simulink model "hpt_v2_1to1_switchlevel"  (R2025a)
settings: Solver=ode23tb  StartTime=0.0  StopTime=0.2  RelTol=1e-3
model workspace (MAT data in the model file):
  hpt_ctrl_Ts = 2e-05
  hpt_energy_bridge_polarity = -1
  hpt_energy_control_sign = -1
  hpt_energy_i_ki = 100
  hpt_energy_i_kp = 0.5
  hpt_energy_id_max = 20
  hpt_energy_openloop_amp = 0
  hpt_energy_openloop_phase = 0
  hpt_energy_vff_gain = 1.06
  hpt_grid_f0 = 50
  hpt_inj_phase_offset = -1.05
  hpt_m_energy = 0
  hpt_m_energy_max = 0.95
  hpt_m_reg = 0.1
  hpt_m_reg_max = 0.8
  hpt_pll_ki = 2500
  hpt_pll_kp = 80
  hpt_pwm_fs = 2000
  hpt_sac_actor_select_mode = 0
  hpt_sac_dynamic_reg_limit = 0.8
  hpt_sac_enable = 0
  hpt_sac_energy_enable = 0
  hpt_sac_energy_max = 0.95
  hpt_sac_fixed_energy_d = 0
  hpt_sac_fixed_energy_q = 0
  hpt_sac_fixed_reg_d = 0
  hpt_sac_fixed_reg_q = 0
  hpt_sac_guard_enable = 0
  hpt_sac_i_base_peak = 816.496580928
  hpt_sac_policy_mode = 0
  hpt_sac_reg_d_gain = 1
  hpt_sac_reg_max = 0.8
  hpt_sac_reg_polarity = 1
  hpt_sac_reg_q_gain = 0
  hpt_sac_topology_id = 1
  hpt_sac_vdc_ref = 800
  hpt_sac_vref_phase = 230
  hpt_swell_gain_scale = 1
  hpt_vdc_ki = 0.2
  hpt_vdc_kp = 0.1
  hpt_vdc_ref = 800
  hpt_vref_lv = 207
  hpt_vreg_ki = 0
  hpt_vreg_kp = 20
libraries: simulink x9, spsLinearTransformerLib x9, spsUniversalBridgeLib x4, spsGroundLib x4, spsThreePhaseVIMeasurementLib x3, spsSeriesRLCBranchLib x2, spsThreePhaseSeriesRLCBranchLib x2, spsIGBTLib x1, spsThreePhaseSourceLib x1, spsThreePhaseSeriesRLCLoadLib x1, spsVoltageMeasurementLib x1, spspowerguiLib x1
settings Model: Creator=m1391  LastModifiedBy=m1391

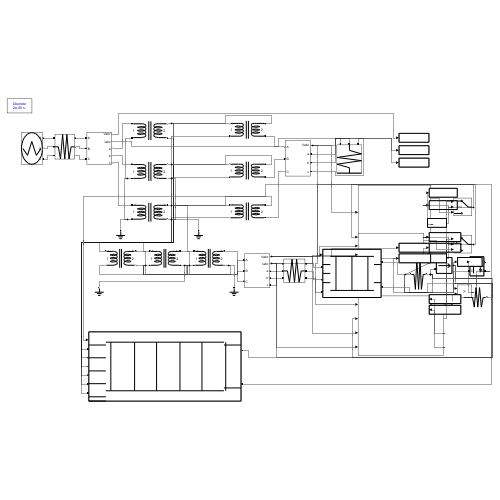
[thumbnail: Simulink's stored preview of the top-level diagram]
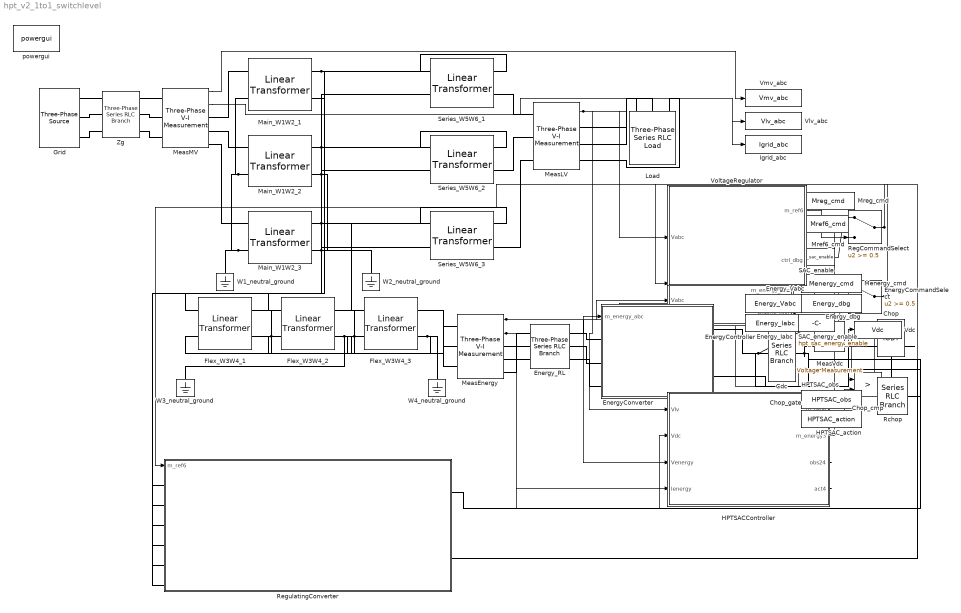
== system hpt_v2_1to1_switchlevel ==
  Cdc : spsSeriesRLCBranchLib/Series RLC Branch  LConnTagsString=__new0  RConnTagsString=__new0  BranchType=C  Resistance=1  Inductance=1e-3  SetiL0=off  InitialCurrent=0  Capacitance=0.0022  Setx0=on  InitialVoltage=800  Measurements=None
  Chop : spsIGBTLib/IGBT  Ron=0.001  Lon=0  Vf=1  Tf=1e-6  Tt=2e-6  IC=0  Rs=1e5  Cs=inf  Measurements=on
  Chop_cmp : RelationalOperator  Operator=>  OutDataTypeStr=boolean  RndMeth=Simplest  InputSameDT=off
  Chop_gate : Constant  Value=850
      mask Display: plot([20 80 80 20 20],[30 30 70 70 30]);
  EnergyCommandSelect : Switch  Threshold=0.5  SaturateOnIntegerOverflow=off  InputSameDT=off
  EnergyController : Subsystem
  EnergyConverter : Subsystem
      mask Display:
      | color('black');
      | plot([10 90 90 10 10],[10 10 90 90 10]);
      | plot([20 80],[78 78]); plot([20 80],[22 22]);
      | plot([28 28],[22 78]); plot([50 50],[22 78]); plot([72 72],[22 78]);
      | plot([10 20],[65 65]); plot([10 20],[50 50]); plot([10 20],[35 35]);
      | plot([80 90],[65 65]); plot([80 90],[35 35]);
  Energy_Iabc : ToWorkspace  VariableName=Energy_Iabc  SampleTime=2e-05
      mask Display: plot([10 90 90 10 10],[25 25 75 75 25]);
  Energy_RL : spsThreePhaseSeriesRLCBranchLib/Three-Phase Series RLC Branch  LConnTagsString=A|B|C  RConnTagsString=A|B|C  BranchType=RL  Resistance=0.05  Inductance=0.003  Capacitance=1e-6  Measurements=None
  Energy_Vabc : ToWorkspace  VariableName=Energy_Vabc  SampleTime=2e-05
      mask Display: plot([10 90 90 10 10],[25 25 75 75 25]);
  Energy_dbg : ToWorkspace  VariableName=Energy_dbg  SampleTime=2e-05
      mask Display: plot([10 90 90 10 10],[25 25 75 75 25]);
  Flex_W3W4_1 : spsLinearTransformerLib/Linear Transformer  UNITS=pu  NominalPower=[40000,50]  winding1=[230.9401,0.005,0.02]  winding2=[230.9401,0.005,0.02]  ThreeWindings=off  winding3=[ 315e3 0.002 0.08 ]  RmLm=[ 500 500 ]  Measurements=None  DataType=off
  Flex_W3W4_2 : spsLinearTransformerLib/Linear Transformer  UNITS=pu  NominalPower=[40000,50]  winding1=[230.9401,0.005,0.02]  winding2=[230.9401,0.005,0.02]  ThreeWindings=off  winding3=[ 315e3 0.002 0.08 ]  RmLm=[ 500 500 ]  Measurements=None  DataType=off
  Flex_W3W4_3 : spsLinearTransformerLib/Linear Transformer  UNITS=pu  NominalPower=[40000,50]  winding1=[230.9401,0.005,0.02]  winding2=[230.9401,0.005,0.02]  ThreeWindings=off  winding3=[ 315e3 0.002 0.08 ]  RmLm=[ 500 500 ]  Measurements=None  DataType=off
  Grid : spsThreePhaseSourceLib/Three-Phase Source  InternalConnection=Yg  VoltagePhases=off  Voltage=10000  PhaseAngle=0  Voltage_phases=[25e3 25e3 25e3]/sqrt(3)  PhaseAngles_phases=[0 -120 +120]  Frequency=50  NonIdealSource=on  SpecifyImpedance=off  Resistance=1e-3  Inductance=1e-5  ShortCircuitLevel=100e6  BaseVoltage=25e3  XRratio=7  BusType=swing  Pref=10e3  Qref=0  Prefabc=[10e3, 10e3, 10e3]  Qrefabc=[0, 0, 0]  Qmin=-inf  Qmax=inf
  HPTSACController : Subsystem
  HPTSAC_action : ToWorkspace  VariableName=HPTSAC_action  SampleTime=2e-05
      mask Display: plot([10 90 90 10 10],[25 25 75 75 25]);
  HPTSAC_obs : ToWorkspace  VariableName=HPTSAC_obs  SampleTime=2e-05
      mask Display: plot([10 90 90 10 10],[25 25 75 75 25]);
  Igrid_abc : ToWorkspace  VariableName=Igrid_abc  SampleTime=2e-05
      mask Display: plot([10 90 90 10 10],[25 25 75 75 25]);
  Load : spsThreePhaseSeriesRLCLoadLib/Three-Phase Series RLC Load  LConnTagsString=A|B|C  Configuration=Y (grounded)  NominalVoltage=400  Vabc=[1e3 1e3 1e3]  Vabcp=[1e3 1e3 1e3]  NominalFrequency=50  UnbalancedPower=off  ActivePower=400000  InductivePower=0  CapacitivePower=0  Pabc=[10e3 9e3 11e3]  QLabc=[100 90 110]  QCabc=[100 90 110]  Pabcp=[10e3 9e3 11e3]  QLabcp=[100 90 110]  QCabcp=[100 90 110]  Measurements=None  LoadType=constant Z
  Main_W1W2_1 : spsLinearTransformerLib/Linear Transformer  UNITS=pu  NominalPower=[133333.3333,50]  winding1=[5773.5027,0.005,0.025]  winding2=[230.9401,0.005,0.025]  ThreeWindings=off  winding3=[ 315e3 0.002 0.08 ]  RmLm=[ 500 500 ]  Measurements=None  DataType=off
  Main_W1W2_2 : spsLinearTransformerLib/Linear Transformer  UNITS=pu  NominalPower=[133333.3333,50]  winding1=[5773.5027,0.005,0.025]  winding2=[230.9401,0.005,0.025]  ThreeWindings=off  winding3=[ 315e3 0.002 0.08 ]  RmLm=[ 500 500 ]  Measurements=None  DataType=off
  Main_W1W2_3 : spsLinearTransformerLib/Linear Transformer  UNITS=pu  NominalPower=[133333.3333,50]  winding1=[5773.5027,0.005,0.025]  winding2=[230.9401,0.005,0.025]  ThreeWindings=off  winding3=[ 315e3 0.002 0.08 ]  RmLm=[ 500 500 ]  Measurements=None  DataType=off
  MeasEnergy : spsThreePhaseVIMeasurementLib/Three-Phase V-I Measurement  VoltageMeasurement=phase-to-ground  SetLabelV=off  LabelV=Vabc  Vpu=off  VpuLL=off  CurrentMeasurement=yes  SetLabelI=off  LabelI=Iabc  Ipu=off  Pbase=100e6  Vbase=500e3  OutputType=Complex  PhasorSimulation=off  PSBequivalent=0
  MeasLV : spsThreePhaseVIMeasurementLib/Three-Phase V-I Measurement  VoltageMeasurement=phase-to-ground  SetLabelV=off  LabelV=Vabc  Vpu=off  VpuLL=off  CurrentMeasurement=no  SetLabelI=off  LabelI=Iabc  Ipu=off  Pbase=100e6  Vbase=500e3  OutputType=Complex  PhasorSimulation=off  PSBequivalent=0
  MeasMV : spsThreePhaseVIMeasurementLib/Three-Phase V-I Measurement  VoltageMeasurement=phase-to-ground  SetLabelV=off  LabelV=Vabc  Vpu=off  VpuLL=off  CurrentMeasurement=yes  SetLabelI=off  LabelI=Iabc  Ipu=off  Pbase=100e6  Vbase=500e3  OutputType=Complex  PhasorSimulation=off  PSBequivalent=0
  MeasVdc : spsVoltageMeasurementLib/Voltage Measurement  PhasorSimulation=off  OutputType=Complex  PSBequivalent=0
  Menergy_cmd : ToWorkspace  VariableName=Menergy_cmd  SampleTime=2e-05
      mask Display: plot([10 90 90 10 10],[25 25 75 75 25]);
  Mref6_cmd : ToWorkspace  VariableName=Mref6_cmd  SampleTime=2e-05
      mask Display: plot([10 90 90 10 10],[25 25 75 75 25]);
  Mreg_cmd : ToWorkspace  VariableName=Mreg_cmd  SampleTime=2e-05
      mask Display: plot([10 90 90 10 10],[25 25 75 75 25]);
  Rchop : spsSeriesRLCBranchLib/Series RLC Branch  LConnTagsString=__new0  RConnTagsString=__new0  BranchType=R  Resistance=5.3333  Inductance=1e-3  SetiL0=off  InitialCurrent=0  Capacitance=1e-6  Setx0=off  InitialVoltage=0  Measurements=None
  RegCommandSelect : Switch  Threshold=0.5  SaturateOnIntegerOverflow=off  InputSameDT=off
  RegulatingConverter : Subsystem
      mask Display:
      | color('black');
      | plot([5 95 95 5 5],[10 10 90 90 10]);
      | plot([15 85],[78 78]); plot([15 85],[22 22]);
      | plot([18 18],[22 78]); plot([32 32],[22 78]);
      | plot([45 45],[22 78]); plot([59 59],[22 78]);
      | plot([72 72],[22 78]); plot([86 86],[22 78]);
      | plot([5 15],[75 75]); plot([5 15],[60 60]); plot([5 15],[45 45]);
      | plot([5 15],[30 30]); plot([5 15],[15 15]); plot([5 15],[10 10]);
      | plot([85 95],[75 75]); plot([85 95],[25 25]);
  SAC_enable : Constant  Value=hpt_sac_enable
      mask Display: plot([20 80 80 20 20],[30 30 70 70 30]);
  SAC_energy_enable : Constant  Value=hpt_sac_energy_enable
      mask Display: plot([20 80 80 20 20],[30 30 70 70 30]);
  Series_W5W6_1 : spsLinearTransformerLib/Linear Transformer  UNITS=pu  NominalPower=[30000,50]  winding1=[400,0.002,0.03]  winding2=[100,0.002,0.03]  ThreeWindings=off  winding3=[ 315e3 0.002 0.08 ]  RmLm=[ 500 500 ]  Measurements=None  DataType=off
  Series_W5W6_2 : spsLinearTransformerLib/Linear Transformer  UNITS=pu  NominalPower=[30000,50]  winding1=[400,0.002,0.03]  winding2=[100,0.002,0.03]  ThreeWindings=off  winding3=[ 315e3 0.002 0.08 ]  RmLm=[ 500 500 ]  Measurements=None  DataType=off
  Series_W5W6_3 : spsLinearTransformerLib/Linear Transformer  UNITS=pu  NominalPower=[30000,50]  winding1=[400,0.002,0.03]  winding2=[100,0.002,0.03]  ThreeWindings=off  winding3=[ 315e3 0.002 0.08 ]  RmLm=[ 500 500 ]  Measurements=None  DataType=off
  Vdc : ToWorkspace  VariableName=Vdc  SampleTime=2e-05
      mask Display: plot([10 90 90 10 10],[25 25 75 75 25]);
  Vlv_abc : ToWorkspace  VariableName=Vlv_abc  SampleTime=2e-05
      mask Display: plot([10 90 90 10 10],[25 25 75 75 25]);
  Vmv_abc : ToWorkspace  VariableName=Vmv_abc  SampleTime=2e-05
      mask Display: plot([10 90 90 10 10],[25 25 75 75 25]);
  VoltageRegulator : Subsystem
  W1_neutral_ground : spsGroundLib/Ground  LConnTagsString=a
  W2_neutral_ground : spsGroundLib/Ground  LConnTagsString=a
  W3_neutral_ground : spsGroundLib/Ground  LConnTagsString=a
  W4_neutral_ground : spsGroundLib/Ground  LConnTagsString=a
  Zg : spsThreePhaseSeriesRLCBranchLib/Three-Phase Series RLC Branch  LConnTagsString=A|B|C  RConnTagsString=A|B|C  BranchType=RL  Resistance=11.7851  Inductance=0.26259  Capacitance=1e-6  Measurements=None
  powergui : spspowerguiLib/powergui  Priority=1  SimulationMode=Discrete  SampleTime=2e-05  frequency=60  Iterations=50  frequencyindice=60  Pbase=100e6  ErrMax=1e-4  UnitsV=kV  UnitsW=MW  buscounter=0  FunctionMessages=off  echomessages=off  EnableUseOfTLC=off  CurrentSourceSwitches=off  DisableSnubberDevices=off  DisableRonSwitches=off  DisableVfSwitches=off  DisplayEquations=off  AutomaticDiscreteSolvers=off  SolverType=Tustin/Backward Euler (TBE)  Interpol=off  ExternalGateDelay=off  methode=off  Ts=100  x0status=blocks  SPID=on  SwTol=0  HookPort=off  NonlinearTolerance=1e-4  nMaxIteration=100  ContinueOnMaxIteration=off  RestoreLinks=warning  ResistiveCurrentMeasurement=off  Frange=[0:2:500]  Ylog=off  Xlog=on  ShowGrid=off  save=off  variable=ZData  structure=0  ZoomFFT=off  StartTime=0.0  cycles=1  DisplayStyle=1  fundamental=60  FreqAxis=off  MaxFrequency=1000  frequencyindicesteady=1  RmsSteady=1  display=off
  wires:
  MeasVdc/1 -> Chop_cmp/1, Vdc/1, HPTSACController/2(Vdc), EnergyController/1(Vdc)
  Chop_gate/1 -> Chop_cmp/2
  Chop_cmp/1 -> Chop/1
  MeasMV/1 -> Vmv_abc/1
  MeasMV/2 -> Igrid_abc/1
  MeasLV/1 -> Vlv_abc/1, VoltageRegulator/1(Vabc), HPTSACController/1(Vlv)
  VoltageRegulator/1(m_ref6) -> RegCommandSelect/3
  HPTSACController/1(m_reg6) -> RegCommandSelect/1
  SAC_enable/1 -> RegCommandSelect/2
  RegCommandSelect/1 -> RegulatingConverter/1(m_ref6), Mref6_cmd/1
  VoltageRegulator/2(ctrl_dbg) -> Mreg_cmd/1
  MeasEnergy/1 -> EnergyController/2(Vabc), HPTSACController/3(Venergy), Energy_Vabc/1
  MeasEnergy/2 -> EnergyController/3(Iabc), HPTSACController/4(Ienergy), Energy_Iabc/1
  EnergyController/1(m_energy_abc) -> EnergyCommandSelect/3
  HPTSACController/2(m_energy3) -> EnergyCommandSelect/1
  SAC_energy_enable/1 -> EnergyCommandSelect/2
  EnergyCommandSelect/1 -> EnergyConverter/1(m_energy_abc), Menergy_cmd/1
  EnergyController/2(energy_dbg) -> Energy_dbg/1
  HPTSACController/3(obs24) -> HPTSAC_obs/1
  HPTSACController/4(act4) -> HPTSAC_action/1
  connections:
  Grid/RConn1 -- Zg/LConn1
  Zg/RConn1 -- MeasMV/LConn1
  MeasMV/RConn1 -- Main_W1W2_1/LConn1
  Series_W5W6_1/RConn1 -- Main_W1W2_1/RConn1 -- Flex_W3W4_1/LConn1
  Series_W5W6_1/RConn2 -- MeasLV/LConn1
  MeasLV/RConn1 -- Load/LConn1
  Flex_W3W4_1/RConn1 -- MeasEnergy/LConn1
  MeasEnergy/RConn1 -- Energy_RL/LConn1
  Energy_RL/RConn1 -- EnergyConverter/LConn1
  Series_W5W6_1/LConn1 -- RegulatingConverter/LConn1
  Series_W5W6_1/LConn2 -- RegulatingConverter/LConn2
  Grid/RConn2 -- Zg/LConn2
  Zg/RConn2 -- MeasMV/LConn2
  MeasMV/RConn2 -- Main_W1W2_2/LConn1
  Series_W5W6_2/RConn1 -- Main_W1W2_2/RConn1 -- Flex_W3W4_2/LConn1
  Series_W5W6_2/RConn2 -- MeasLV/LConn2
  MeasLV/RConn2 -- Load/LConn2
  Flex_W3W4_2/RConn1 -- MeasEnergy/LConn2
  MeasEnergy/RConn2 -- Energy_RL/LConn2
  Energy_RL/RConn2 -- EnergyConverter/LConn2
  Series_W5W6_2/LConn1 -- RegulatingConverter/LConn3
  Series_W5W6_2/LConn2 -- RegulatingConverter/LConn4
  Grid/RConn3 -- Zg/LConn3
  Zg/RConn3 -- MeasMV/LConn3
  MeasMV/RConn3 -- Main_W1W2_3/LConn1
  Series_W5W6_3/RConn1 -- Main_W1W2_3/RConn1 -- Flex_W3W4_3/LConn1
  Series_W5W6_3/RConn2 -- MeasLV/LConn3
  MeasLV/RConn3 -- Load/LConn3
  Flex_W3W4_3/RConn1 -- MeasEnergy/LConn3
  MeasEnergy/RConn3 -- Energy_RL/LConn3
  Energy_RL/RConn3 -- EnergyConverter/LConn3
  Series_W5W6_3/LConn1 -- RegulatingConverter/LConn5
  Series_W5W6_3/LConn2 -- RegulatingConverter/LConn6
  Main_W1W2_2/LConn2 -- Main_W1W2_1/LConn2 -- Main_W1W2_3/LConn2 -- W1_neutral_ground/LConn1
  Main_W1W2_2/RConn2 -- Main_W1W2_1/RConn2 -- Main_W1W2_3/RConn2 -- W2_neutral_ground/LConn1
  Flex_W3W4_2/LConn2 -- Flex_W3W4_1/LConn2 -- Flex_W3W4_3/LConn2 -- W3_neutral_ground/LConn1
  Flex_W3W4_2/RConn2 -- Flex_W3W4_1/RConn2 -- Flex_W3W4_3/RConn2 -- W4_neutral_ground/LConn1
  EnergyConverter/RConn1 -- Cdc/LConn1 -- RegulatingConverter/RConn1 -- MeasVdc/LConn1 -- Chop/LConn1
  EnergyConverter/RConn2 -- RegulatingConverter/RConn2 -- MeasVdc/LConn2 -- Cdc/RConn1 -- Rchop/RConn1
  Chop/RConn1 -- Rchop/LConn1

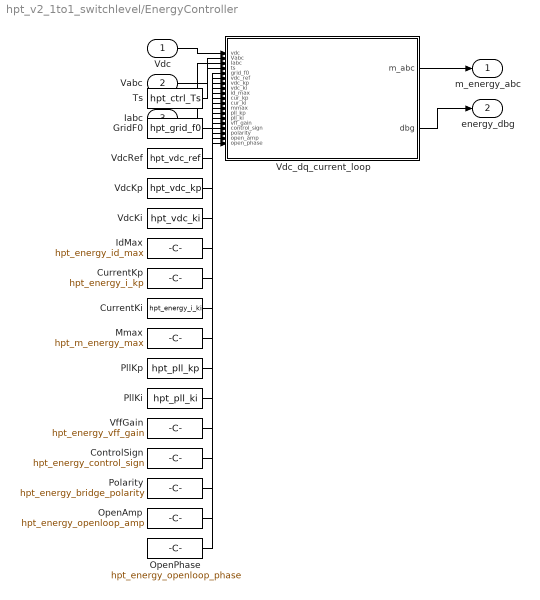
== system hpt_v2_1to1_switchlevel/EnergyController ==
  Vdc : Inport
  Vabc : Inport  Port=2
  Iabc : Inport  Port=3
  ControlSign : Constant  Value=hpt_energy_control_sign
      mask Display: plot([20 80 80 20 20],[30 30 70 70 30]);
  CurrentKi : Constant  Value=hpt_energy_i_ki
      mask Display: plot([20 80 80 20 20],[30 30 70 70 30]);
  CurrentKp : Constant  Value=hpt_energy_i_kp
      mask Display: plot([20 80 80 20 20],[30 30 70 70 30]);
  GridF0 : Constant  Value=hpt_grid_f0
      mask Display: plot([20 80 80 20 20],[30 30 70 70 30]);
  IdMax : Constant  Value=hpt_energy_id_max
      mask Display: plot([20 80 80 20 20],[30 30 70 70 30]);
  Mmax : Constant  Value=hpt_m_energy_max
      mask Display: plot([20 80 80 20 20],[30 30 70 70 30]);
  OpenAmp : Constant  Value=hpt_energy_openloop_amp
      mask Display: plot([20 80 80 20 20],[30 30 70 70 30]);
  OpenPhase : Constant  Value=hpt_energy_openloop_phase
      mask Display: plot([20 80 80 20 20],[30 30 70 70 30]);
  PllKi : Constant  Value=hpt_pll_ki
      mask Display: plot([20 80 80 20 20],[30 30 70 70 30]);
  PllKp : Constant  Value=hpt_pll_kp
      mask Display: plot([20 80 80 20 20],[30 30 70 70 30]);
  Polarity : Constant  Value=hpt_energy_bridge_polarity
      mask Display: plot([20 80 80 20 20],[30 30 70 70 30]);
  Ts : Constant  Value=hpt_ctrl_Ts
      mask Display: plot([20 80 80 20 20],[30 30 70 70 30]);
  VdcKi : Constant  Value=hpt_vdc_ki
      mask Display: plot([20 80 80 20 20],[30 30 70 70 30]);
  VdcKp : Constant  Value=hpt_vdc_kp
      mask Display: plot([20 80 80 20 20],[30 30 70 70 30]);
  VdcRef : Constant  Value=hpt_vdc_ref
      mask Display: plot([20 80 80 20 20],[30 30 70 70 30]);
  Vdc_dq_current_loop : MATLAB Function  TreatAsAtomicUnit=on
  VffGain : Constant  Value=hpt_energy_vff_gain
      mask Display: plot([20 80 80 20 20],[30 30 70 70 30]);
  m_energy_abc : Outport
  energy_dbg : Outport  Port=2
  wires:
  Ts/1 -> Vdc_dq_current_loop/4(ts)
  GridF0/1 -> Vdc_dq_current_loop/5(grid_f0)
  VdcRef/1 -> Vdc_dq_current_loop/6(vdc_ref)
  VdcKp/1 -> Vdc_dq_current_loop/7(vdc_kp)
  VdcKi/1 -> Vdc_dq_current_loop/8(vdc_ki)
  IdMax/1 -> Vdc_dq_current_loop/9(id_max)
  CurrentKp/1 -> Vdc_dq_current_loop/10(cur_kp)
  CurrentKi/1 -> Vdc_dq_current_loop/11(cur_ki)
  Mmax/1 -> Vdc_dq_current_loop/12(mmax)
  PllKp/1 -> Vdc_dq_current_loop/13(pll_kp)
  PllKi/1 -> Vdc_dq_current_loop/14(pll_ki)
  VffGain/1 -> Vdc_dq_current_loop/15(vff_gain)
  ControlSign/1 -> Vdc_dq_current_loop/16(control_sign)
  Polarity/1 -> Vdc_dq_current_loop/17(polarity)
  OpenAmp/1 -> Vdc_dq_current_loop/18(open_amp)
  OpenPhase/1 -> Vdc_dq_current_loop/19(open_phase)
  Vdc/1 -> Vdc_dq_current_loop/1(vdc)
  Vabc/1 -> Vdc_dq_current_loop/2(Vabc)
  Iabc/1 -> Vdc_dq_current_loop/3(Iabc)
  Vdc_dq_current_loop/1(m_abc) -> m_energy_abc/1
  Vdc_dq_current_loop/2(dbg) -> energy_dbg/1

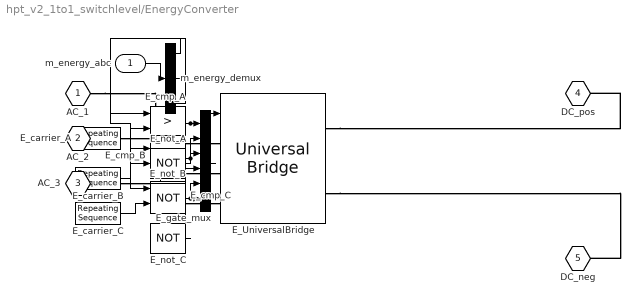
== system hpt_v2_1to1_switchlevel/EnergyConverter ==
  m_energy_abc : Inport
  E_UniversalBridge : spsUniversalBridgeLib/Universal Bridge  Arms=3  SnubberResistance=1e5  SnubberCapacitance=inf  Device=IGBT / Diodes  Ron=1e-3  Lon=0  ForwardVoltages=[0.8 0.8]  ForwardVoltage=0  GTOparameters=[ 10e-6 , 20e-6 ]  IGBTparameters=[ 1e-6 , 2e-6 ]  Measurements=None  Measurements_2=None  converterType=Rectifier
  E_carrier_A : simulink/Sources/Repeating Sequence  rep_seq_t=[0 0.5/hpt_pwm_fs 1/hpt_pwm_fs]  rep_seq_y=[-1 1 -1]
  E_carrier_B : simulink/Sources/Repeating Sequence  rep_seq_t=[0 0.5/hpt_pwm_fs 1/hpt_pwm_fs]  rep_seq_y=[-1 1 -1]
  E_carrier_C : simulink/Sources/Repeating Sequence  rep_seq_t=[0 0.5/hpt_pwm_fs 1/hpt_pwm_fs]  rep_seq_y=[-1 1 -1]
  E_cmp_A : RelationalOperator  Operator=>  OutDataTypeStr=boolean  RndMeth=Simplest  InputSameDT=off
  E_cmp_B : RelationalOperator  Operator=>  OutDataTypeStr=boolean  RndMeth=Simplest  InputSameDT=off
  E_cmp_C : RelationalOperator  Operator=>  OutDataTypeStr=boolean  RndMeth=Simplest  InputSameDT=off
  E_gate_mux : Mux  Inputs=6
  E_not_A : Logic  Operator=NOT  AllPortsSameDT=off  OutDataTypeStr=boolean
  E_not_B : Logic  Operator=NOT  AllPortsSameDT=off  OutDataTypeStr=boolean
  E_not_C : Logic  Operator=NOT  AllPortsSameDT=off  OutDataTypeStr=boolean
  m_energy_demux : Demux  Outputs=3
  AC_1 : PMIOPort  Side=Left
  AC_2 : PMIOPort  Port=2  Side=Left
  AC_3 : PMIOPort  Port=3  Side=Left
  DC_pos : PMIOPort  Port=4  Side=Right
  DC_neg : PMIOPort  Port=5  Side=Right
  wires:
  m_energy_abc/1 -> m_energy_demux/1
  m_energy_demux/1 -> E_cmp_A/1
  E_carrier_A/1 -> E_cmp_A/2
  E_cmp_A/1 -> E_gate_mux/1, E_not_A/1
  E_not_A/1 -> E_gate_mux/2
  m_energy_demux/2 -> E_cmp_B/1
  E_carrier_B/1 -> E_cmp_B/2
  E_cmp_B/1 -> E_gate_mux/3, E_not_B/1
  E_not_B/1 -> E_gate_mux/4
  m_energy_demux/3 -> E_cmp_C/1
  E_carrier_C/1 -> E_cmp_C/2
  E_cmp_C/1 -> E_gate_mux/5, E_not_C/1
  E_not_C/1 -> E_gate_mux/6
  E_gate_mux/1 -> E_UniversalBridge/1
  connections:
  AC_1/RConn1 -- E_UniversalBridge/LConn1
  AC_2/RConn1 -- E_UniversalBridge/LConn2
  AC_3/RConn1 -- E_UniversalBridge/LConn3
  E_UniversalBridge/RConn1 -- DC_pos/RConn1
  E_UniversalBridge/RConn2 -- DC_neg/RConn1

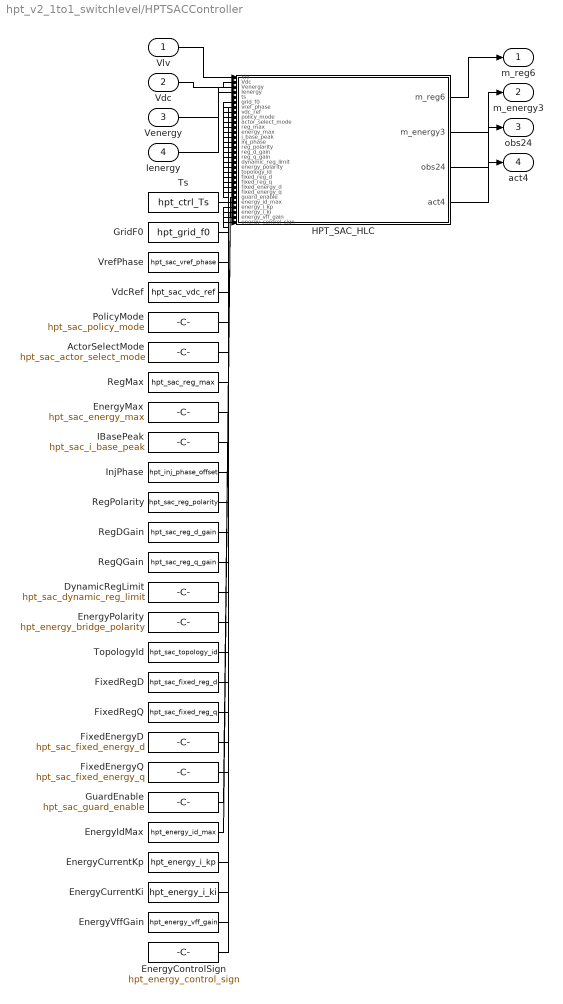
== system hpt_v2_1to1_switchlevel/HPTSACController ==
  Vlv : Inport
  Vdc : Inport  Port=2
  Venergy : Inport  Port=3
  Ienergy : Inport  Port=4
  ActorSelectMode : Constant  Value=hpt_sac_actor_select_mode
      mask Display: plot([20 80 80 20 20],[30 30 70 70 30]);
  DynamicRegLimit : Constant  Value=hpt_sac_dynamic_reg_limit
      mask Display: plot([20 80 80 20 20],[30 30 70 70 30]);
  EnergyControlSign : Constant  Value=hpt_energy_control_sign
      mask Display: plot([20 80 80 20 20],[30 30 70 70 30]);
  EnergyCurrentKi : Constant  Value=hpt_energy_i_ki
      mask Display: plot([20 80 80 20 20],[30 30 70 70 30]);
  EnergyCurrentKp : Constant  Value=hpt_energy_i_kp
      mask Display: plot([20 80 80 20 20],[30 30 70 70 30]);
  EnergyIdMax : Constant  Value=hpt_energy_id_max
      mask Display: plot([20 80 80 20 20],[30 30 70 70 30]);
  EnergyMax : Constant  Value=hpt_sac_energy_max
      mask Display: plot([20 80 80 20 20],[30 30 70 70 30]);
  EnergyPolarity : Constant  Value=hpt_energy_bridge_polarity
      mask Display: plot([20 80 80 20 20],[30 30 70 70 30]);
  EnergyVffGain : Constant  Value=hpt_energy_vff_gain
      mask Display: plot([20 80 80 20 20],[30 30 70 70 30]);
  FixedEnergyD : Constant  Value=hpt_sac_fixed_energy_d
      mask Display: plot([20 80 80 20 20],[30 30 70 70 30]);
  FixedEnergyQ : Constant  Value=hpt_sac_fixed_energy_q
      mask Display: plot([20 80 80 20 20],[30 30 70 70 30]);
  FixedRegD : Constant  Value=hpt_sac_fixed_reg_d
      mask Display: plot([20 80 80 20 20],[30 30 70 70 30]);
  FixedRegQ : Constant  Value=hpt_sac_fixed_reg_q
      mask Display: plot([20 80 80 20 20],[30 30 70 70 30]);
  GridF0 : Constant  Value=hpt_grid_f0
      mask Display: plot([20 80 80 20 20],[30 30 70 70 30]);
  GuardEnable : Constant  Value=hpt_sac_guard_enable
      mask Display: plot([20 80 80 20 20],[30 30 70 70 30]);
  HPT_SAC_HLC : MATLAB Function  TreatAsAtomicUnit=on
  IBasePeak : Constant  Value=hpt_sac_i_base_peak
      mask Display: plot([20 80 80 20 20],[30 30 70 70 30]);
  InjPhase : Constant  Value=hpt_inj_phase_offset
      mask Display: plot([20 80 80 20 20],[30 30 70 70 30]);
  PolicyMode : Constant  Value=hpt_sac_policy_mode
      mask Display: plot([20 80 80 20 20],[30 30 70 70 30]);
  RegDGain : Constant  Value=hpt_sac_reg_d_gain
      mask Display: plot([20 80 80 20 20],[30 30 70 70 30]);
  RegMax : Constant  Value=hpt_sac_reg_max
      mask Display: plot([20 80 80 20 20],[30 30 70 70 30]);
  RegPolarity : Constant  Value=hpt_sac_reg_polarity
      mask Display: plot([20 80 80 20 20],[30 30 70 70 30]);
  RegQGain : Constant  Value=hpt_sac_reg_q_gain
      mask Display: plot([20 80 80 20 20],[30 30 70 70 30]);
  TopologyId : Constant  Value=hpt_sac_topology_id
      mask Display: plot([20 80 80 20 20],[30 30 70 70 30]);
  Ts : Constant  Value=hpt_ctrl_Ts
      mask Display: plot([20 80 80 20 20],[30 30 70 70 30]);
  VdcRef : Constant  Value=hpt_sac_vdc_ref
      mask Display: plot([20 80 80 20 20],[30 30 70 70 30]);
  VrefPhase : Constant  Value=hpt_sac_vref_phase
      mask Display: plot([20 80 80 20 20],[30 30 70 70 30]);
  m_reg6 : Outport
  m_energy3 : Outport  Port=2
  obs24 : Outport  Port=3
  act4 : Outport  Port=4
  wires:
  Ts/1 -> HPT_SAC_HLC/5(ts)
  GridF0/1 -> HPT_SAC_HLC/6(grid_f0)
  VrefPhase/1 -> HPT_SAC_HLC/7(vref_phase)
  VdcRef/1 -> HPT_SAC_HLC/8(vdc_ref)
  PolicyMode/1 -> HPT_SAC_HLC/9(policy_mode)
  ActorSelectMode/1 -> HPT_SAC_HLC/10(actor_select_mode)
  RegMax/1 -> HPT_SAC_HLC/11(reg_max)
  EnergyMax/1 -> HPT_SAC_HLC/12(energy_max)
  IBasePeak/1 -> HPT_SAC_HLC/13(i_base_peak)
  InjPhase/1 -> HPT_SAC_HLC/14(inj_phase)
  RegPolarity/1 -> HPT_SAC_HLC/15(reg_polarity)
  RegDGain/1 -> HPT_SAC_HLC/16(reg_d_gain)
  RegQGain/1 -> HPT_SAC_HLC/17(reg_q_gain)
  DynamicRegLimit/1 -> HPT_SAC_HLC/18(dynamic_reg_limit)
  EnergyPolarity/1 -> HPT_SAC_HLC/19(energy_polarity)
  TopologyId/1 -> HPT_SAC_HLC/20(topology_id)
  FixedRegD/1 -> HPT_SAC_HLC/21(fixed_reg_d)
  FixedRegQ/1 -> HPT_SAC_HLC/22(fixed_reg_q)
  FixedEnergyD/1 -> HPT_SAC_HLC/23(fixed_energy_d)
  FixedEnergyQ/1 -> HPT_SAC_HLC/24(fixed_energy_q)
  GuardEnable/1 -> HPT_SAC_HLC/25(guard_enable)
  EnergyIdMax/1 -> HPT_SAC_HLC/26(energy_id_max)
  EnergyCurrentKp/1 -> HPT_SAC_HLC/27(energy_i_kp)
  EnergyCurrentKi/1 -> HPT_SAC_HLC/28(energy_i_ki)
  EnergyVffGain/1 -> HPT_SAC_HLC/29(energy_vff_gain)
  EnergyControlSign/1 -> HPT_SAC_HLC/30(energy_control_sign)
  Vlv/1 -> HPT_SAC_HLC/1(Vlv)
  Vdc/1 -> HPT_SAC_HLC/2(Vdc)
  Venergy/1 -> HPT_SAC_HLC/3(Venergy)
  Ienergy/1 -> HPT_SAC_HLC/4(Ienergy)
  HPT_SAC_HLC/1(m_reg6) -> m_reg6/1
  HPT_SAC_HLC/2(m_energy3) -> m_energy3/1
  HPT_SAC_HLC/3(obs24) -> obs24/1
  HPT_SAC_HLC/4(act4) -> act4/1

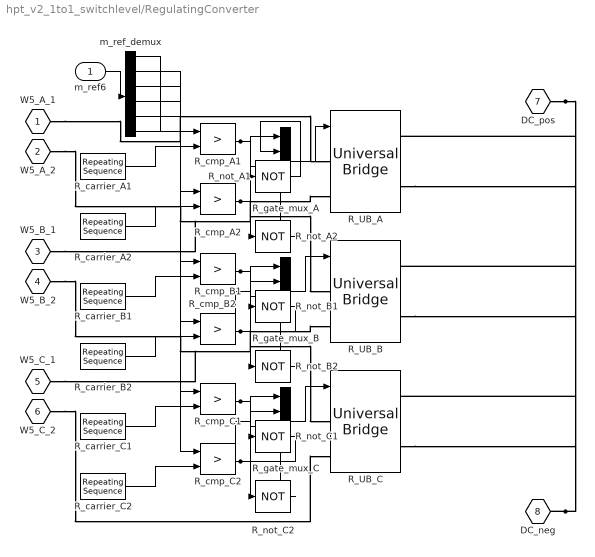
== system hpt_v2_1to1_switchlevel/RegulatingConverter ==
  m_ref6 : Inport
  R_UB_A : spsUniversalBridgeLib/Universal Bridge  Arms=2  SnubberResistance=1e5  SnubberCapacitance=1e-9  Device=IGBT / Diodes  Ron=1e-3  Lon=0  ForwardVoltages="[  0  0  ]"  ForwardVoltage=0  GTOparameters=[ 10e-6 , 20e-6 ]  IGBTparameters=[ 1e-6 , 2e-6 ]  Measurements=None  Measurements_2=None  converterType=Rectifier
  R_UB_B : spsUniversalBridgeLib/Universal Bridge  Arms=2  SnubberResistance=1e5  SnubberCapacitance=1e-9  Device=IGBT / Diodes  Ron=1e-3  Lon=0  ForwardVoltages="[  0  0  ]"  ForwardVoltage=0  GTOparameters=[ 10e-6 , 20e-6 ]  IGBTparameters=[ 1e-6 , 2e-6 ]  Measurements=None  Measurements_2=None  converterType=Rectifier
  R_UB_C : spsUniversalBridgeLib/Universal Bridge  Arms=2  SnubberResistance=1e5  SnubberCapacitance=1e-9  Device=IGBT / Diodes  Ron=1e-3  Lon=0  ForwardVoltages="[  0  0  ]"  ForwardVoltage=0  GTOparameters=[ 10e-6 , 20e-6 ]  IGBTparameters=[ 1e-6 , 2e-6 ]  Measurements=None  Measurements_2=None  converterType=Rectifier
  R_carrier_A1 : simulink/Sources/Repeating Sequence  rep_seq_t=[0 0.5/hpt_pwm_fs 1/hpt_pwm_fs]  rep_seq_y=[-1 1 -1]
  R_carrier_A2 : simulink/Sources/Repeating Sequence  rep_seq_t=[0 0.5/hpt_pwm_fs 1/hpt_pwm_fs]  rep_seq_y=[-1 1 -1]
  R_carrier_B1 : simulink/Sources/Repeating Sequence  rep_seq_t=[0 0.5/hpt_pwm_fs 1/hpt_pwm_fs]  rep_seq_y=[-1 1 -1]
  R_carrier_B2 : simulink/Sources/Repeating Sequence  rep_seq_t=[0 0.5/hpt_pwm_fs 1/hpt_pwm_fs]  rep_seq_y=[-1 1 -1]
  R_carrier_C1 : simulink/Sources/Repeating Sequence  rep_seq_t=[0 0.5/hpt_pwm_fs 1/hpt_pwm_fs]  rep_seq_y=[-1 1 -1]
  R_carrier_C2 : simulink/Sources/Repeating Sequence  rep_seq_t=[0 0.5/hpt_pwm_fs 1/hpt_pwm_fs]  rep_seq_y=[-1 1 -1]
  R_cmp_A1 : RelationalOperator  Operator=>  OutDataTypeStr=boolean  RndMeth=Simplest  InputSameDT=off
  R_cmp_A2 : RelationalOperator  Operator=>  OutDataTypeStr=boolean  RndMeth=Simplest  InputSameDT=off
  R_cmp_B1 : RelationalOperator  Operator=>  OutDataTypeStr=boolean  RndMeth=Simplest  InputSameDT=off
  R_cmp_B2 : RelationalOperator  Operator=>  OutDataTypeStr=boolean  RndMeth=Simplest  InputSameDT=off
  R_cmp_C1 : RelationalOperator  Operator=>  OutDataTypeStr=boolean  RndMeth=Simplest  InputSameDT=off
  R_cmp_C2 : RelationalOperator  Operator=>  OutDataTypeStr=boolean  RndMeth=Simplest  InputSameDT=off
  R_gate_mux_A : Mux
  R_gate_mux_B : Mux
  R_gate_mux_C : Mux
  R_not_A1 : Logic  Operator=NOT  AllPortsSameDT=off  OutDataTypeStr=boolean
  R_not_A2 : Logic  Operator=NOT  AllPortsSameDT=off  OutDataTypeStr=boolean
  R_not_B1 : Logic  Operator=NOT  AllPortsSameDT=off  OutDataTypeStr=boolean
  R_not_B2 : Logic  Operator=NOT  AllPortsSameDT=off  OutDataTypeStr=boolean
  R_not_C1 : Logic  Operator=NOT  AllPortsSameDT=off  OutDataTypeStr=boolean
  R_not_C2 : Logic  Operator=NOT  AllPortsSameDT=off  OutDataTypeStr=boolean
  m_ref_demux : Demux  Outputs=6
  W5_A_1 : PMIOPort  Side=Left
  W5_A_2 : PMIOPort  Port=2  Side=Left
  W5_B_1 : PMIOPort  Port=3  Side=Left
  W5_B_2 : PMIOPort  Port=4  Side=Left
  W5_C_1 : PMIOPort  Port=5  Side=Left
  W5_C_2 : PMIOPort  Port=6  Side=Left
  DC_pos : PMIOPort  Port=7  Side=Right
  DC_neg : PMIOPort  Port=8  Side=Right
  wires:
  m_ref6/1 -> m_ref_demux/1
  m_ref_demux/1 -> R_cmp_A1/1
  R_carrier_A1/1 -> R_cmp_A1/2
  R_cmp_A1/1 -> R_gate_mux_A/1, R_not_A1/1
  R_not_A1/1 -> R_gate_mux_A/2
  m_ref_demux/2 -> R_cmp_A2/1
  R_carrier_A2/1 -> R_cmp_A2/2
  R_cmp_A2/1 -> R_gate_mux_A/3, R_not_A2/1
  R_not_A2/1 -> R_gate_mux_A/4
  R_gate_mux_A/1 -> R_UB_A/1
  m_ref_demux/3 -> R_cmp_B1/1
  R_carrier_B1/1 -> R_cmp_B1/2
  R_cmp_B1/1 -> R_gate_mux_B/1, R_not_B1/1
  R_not_B1/1 -> R_gate_mux_B/2
  m_ref_demux/4 -> R_cmp_B2/1
  R_carrier_B2/1 -> R_cmp_B2/2
  R_cmp_B2/1 -> R_gate_mux_B/3, R_not_B2/1
  R_not_B2/1 -> R_gate_mux_B/4
  R_gate_mux_B/1 -> R_UB_B/1
  m_ref_demux/5 -> R_cmp_C1/1
  R_carrier_C1/1 -> R_cmp_C1/2
  R_cmp_C1/1 -> R_gate_mux_C/1, R_not_C1/1
  R_not_C1/1 -> R_gate_mux_C/2
  m_ref_demux/6 -> R_cmp_C2/1
  R_carrier_C2/1 -> R_cmp_C2/2
  R_cmp_C2/1 -> R_gate_mux_C/3, R_not_C2/1
  R_not_C2/1 -> R_gate_mux_C/4
  R_gate_mux_C/1 -> R_UB_C/1
  connections:
  W5_A_1/RConn1 -- R_UB_A/LConn1
  W5_A_2/RConn1 -- R_UB_A/LConn2
  W5_B_1/RConn1 -- R_UB_B/LConn1
  W5_B_2/RConn1 -- R_UB_B/LConn2
  W5_C_1/RConn1 -- R_UB_C/LConn1
  W5_C_2/RConn1 -- R_UB_C/LConn2
  R_UB_A/RConn1 -- DC_pos/RConn1 -- R_UB_B/RConn1 -- R_UB_C/RConn1
  R_UB_A/RConn2 -- R_UB_B/RConn2 -- DC_neg/RConn1 -- R_UB_C/RConn2

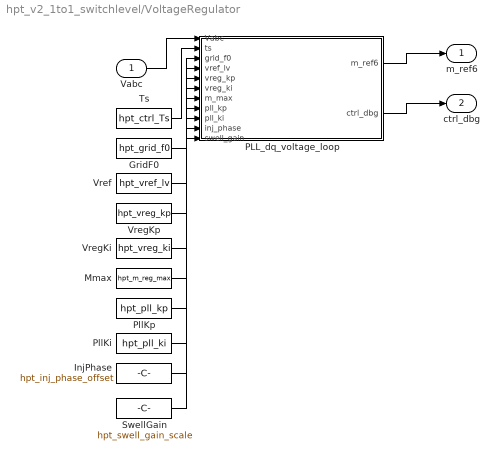
== system hpt_v2_1to1_switchlevel/VoltageRegulator ==
  Vabc : Inport
  GridF0 : Constant  Value=hpt_grid_f0
      mask Display: plot([20 80 80 20 20],[30 30 70 70 30]);
  InjPhase : Constant  Value=hpt_inj_phase_offset
      mask Display: plot([20 80 80 20 20],[30 30 70 70 30]);
  Mmax : Constant  Value=hpt_m_reg_max
      mask Display: plot([20 80 80 20 20],[30 30 70 70 30]);
  PLL_dq_voltage_loop : MATLAB Function  TreatAsAtomicUnit=on
  PllKi : Constant  Value=hpt_pll_ki
      mask Display: plot([20 80 80 20 20],[30 30 70 70 30]);
  PllKp : Constant  Value=hpt_pll_kp
      mask Display: plot([20 80 80 20 20],[30 30 70 70 30]);
  SwellGain : Constant  Value=hpt_swell_gain_scale
      mask Display: plot([20 80 80 20 20],[30 30 70 70 30]);
  Ts : Constant  Value=hpt_ctrl_Ts
      mask Display: plot([20 80 80 20 20],[30 30 70 70 30]);
  Vref : Constant  Value=hpt_vref_lv
      mask Display: plot([20 80 80 20 20],[30 30 70 70 30]);
  VregKi : Constant  Value=hpt_vreg_ki
      mask Display: plot([20 80 80 20 20],[30 30 70 70 30]);
  VregKp : Constant  Value=hpt_vreg_kp
      mask Display: plot([20 80 80 20 20],[30 30 70 70 30]);
  m_ref6 : Outport
  ctrl_dbg : Outport  Port=2
  wires:
  Ts/1 -> PLL_dq_voltage_loop/2(ts)
  GridF0/1 -> PLL_dq_voltage_loop/3(grid_f0)
  Vref/1 -> PLL_dq_voltage_loop/4(vref_lv)
  VregKp/1 -> PLL_dq_voltage_loop/5(vreg_kp)
  VregKi/1 -> PLL_dq_voltage_loop/6(vreg_ki)
  Mmax/1 -> PLL_dq_voltage_loop/7(m_max)
  PllKp/1 -> PLL_dq_voltage_loop/8(pll_kp)
  PllKi/1 -> PLL_dq_voltage_loop/9(pll_ki)
  InjPhase/1 -> PLL_dq_voltage_loop/10(inj_phase)
  SwellGain/1 -> PLL_dq_voltage_loop/11(swell_gain)
  Vabc/1 -> PLL_dq_voltage_loop/1(Vabc)
  PLL_dq_voltage_loop/1(m_ref6) -> m_ref6/1
  PLL_dq_voltage_loop/2(ctrl_dbg) -> ctrl_dbg/1

== matlab function hpt_v2_1to1_switchlevel/EnergyController/Vdc_dq_current_loop ==
  data: vdc input; m_abc output; Vabc input; Iabc input; ts input; grid_f0 input; vdc_ref input; vdc_kp input; vdc_ki input; id_max input; cur_kp input; cur_ki input; mmax input; pll_kp input; pll_ki input; vff_gain input; control_sign input; polarity input; open_amp input; open_phase input; dbg output
function [m_abc, dbg] = fcn(vdc, Vabc, Iabc, ts, grid_f0, vdc_ref, vdc_kp, vdc_ki, id_max, cur_kp, cur_ki, mmax, pll_kp, pll_ki, vff_gain, control_sign, polarity, open_amp, open_phase)
%#codegen
persistent theta xi_pll xi_vdc xi_id xi_iq t_ctrl
if isempty(theta)
    theta = 0;
    xi_pll = 0;
    xi_vdc = 0;
    xi_id = 0;
    xi_iq = 0;
    t_ctrl = 0;
end
t_ctrl = t_ctrl + ts;
va = Vabc(1); vb = Vabc(2); vc = Vabc(3);
ia = Iabc(1); ib = Iabc(2); ic = Iabc(3);
valpha = (2/3) * (va - 0.5*vb - 0.5*vc);
vbeta = (sqrt(3)/3) * (vb - vc);
ialpha = (2/3) * (ia - 0.5*ib - 0.5*ic);
ibeta = (sqrt(3)/3) * (ib - ic);
theta_meas = atan2(vbeta, valpha);
pll_err = atan2(sin(theta_meas - theta), cos(theta_meas - theta));
xi_pll = xi_pll + pll_ki * pll_err * ts;
omega = 2*pi*grid_f0 + pll_kp * pll_err + xi_pll;
theta = theta + omega * ts;
theta = theta - 2*pi*floor(theta/(2*pi));
ct = cos(theta); st = sin(theta);
if open_amp > 0
    mo = min(open_amp, mmax);
    ma = mo * sin(theta + open_phase);
    mb = mo * sin(theta + open_phase - 2*pi/3);
    mc = mo * sin(theta + open_phase + 2*pi/3);
    p_ac = va*ia + vb*ib + vc*ic;
    m_abc = polarity * [ma; mb; mc];
    dbg = [theta; 0; 0; 0; 0; 0; vdc; vdc_ref-vdc; p_ac; ma; mb; mc];
    return;
end
vd = valpha*ct + vbeta*st;
vq = -valpha*st + vbeta*ct;
id = ialpha*ct + ibeta*st;
iq = -ialpha*st + ibeta*ct;
err = vdc_ref - vdc;
if abs(err) < 3 || t_ctrl < 0.02
    xi_vdc = 0;
    id_ref = 0;
else
    xi_vdc = xi_vdc + vdc_ki * err * ts;
    id_unsat = vdc_kp * err + xi_vdc;
    id_ref = min(max(id_unsat, -id_max), id_max);
    if id_ref ~= id_unsat
        xi_vdc = id_ref - vdc_kp * err;
    end
end
iq_ref = 0;
eid = id_ref - id;
eiq = iq_ref - iq;
xi_id = xi_id + cur_ki * eid * ts;
xi_iq = xi_iq + cur_ki * eiq * ts;
vd_ctrl = cur_kp * eid + xi_id;
vq_ctrl = cur_kp * eiq + xi_iq;
vconv_d = vff_gain * vd - control_sign * vd_ctrl;
vconv_q = vff_gain * vq - control_sign * vq_ctrl;
conv_alpha = vconv_d*ct - vconv_q*st;
conv_beta = vconv_d*st + vconv_q*ct;
ma_unsat = 2 * conv_alpha / max(abs(vdc), 50);
mb_unsat = 2 * (-0.5*conv_alpha + (sqrt(3)/2)*conv_beta) / max(abs(vdc), 50);
mc_unsat = 2 * (-0.5*conv_alpha - (sqrt(3)/2)*conv_beta) / max(abs(vdc), 50);
ma = min(max(ma_unsat, -mmax), mmax);
mb = min(max(mb_unsat, -mmax), mmax);
mc = min(max(mc_unsat, -mmax), mmax);
if abs(ma) >= mmax || abs(mb) >= mmax || abs(mc) >= mmax
    xi_id = xi_id - cur_ki * eid * ts;
    xi_iq = xi_iq - cur_ki * eiq * ts;
end
m_abc = polarity * [ma; mb; mc];
p_ac = va*ia + vb*ib + vc*ic;
dbg = [theta; vd; vq; id; iq; id_ref; vdc; err; p_ac; ma; mb; mc];
end

== matlab function hpt_v2_1to1_switchlevel/VoltageRegulator/PLL_dq_voltage_loop ==
  data: Vabc input; m_ref6 output; ts input; grid_f0 input; vref_lv input; vreg_kp input; vreg_ki input; m_max input; pll_kp input; pll_ki input; inj_phase input; swell_gain input; ctrl_dbg output
function [m_ref6, ctrl_dbg] = fcn(Vabc, ts, grid_f0, vref_lv, vreg_kp, vreg_ki, m_max, pll_kp, pll_ki, inj_phase, swell_gain)
%#codegen
persistent theta xi_pll xi_a xi_b xi_c t_ctrl v_rms_f
if isempty(theta)
    theta = 0;
    xi_pll = 0;
    xi_a = 0;
    xi_b = 0;
    xi_c = 0;
    t_ctrl = 0;
    v_rms_f = 0;
end
t_ctrl = t_ctrl + ts;
m_ref6 = zeros(6, 1);
ctrl_dbg = zeros(7, 1);
va = Vabc(1);
vb = Vabc(2);
vc = Vabc(3);
alpha = (2/3) * (va - 0.5*vb - 0.5*vc);
beta = (sqrt(3)/3) * (vb - vc);
theta_meas = atan2(beta, alpha);
pll_err = atan2(sin(theta_meas - theta), cos(theta_meas - theta));
xi_pll = xi_pll + pll_ki * pll_err * ts;
omega = 2*pi*grid_f0 + pll_kp * pll_err + xi_pll;
theta = theta + omega * ts;
theta = theta - 2*pi*floor(theta/(2*pi));
ct = cos(theta);
st = sin(theta);
vd = alpha*ct + beta*st;
vq = -alpha*st + beta*ct;
v_rms = sqrt(max((va*va + vb*vb + vc*vc) / 3, 0));
if v_rms_f == 0
    v_rms_f = v_rms;
end
alpha_v = min(max(ts / 0.005, 0), 1);
v_rms_f = v_rms_f + alpha_v * (v_rms - v_rms_f);
v_meas = v_rms_f;
v_err = vref_lv - v_meas;
err_pu = v_err / max(vref_lv, 1e-6);
phi = inj_phase;
if abs(err_pu) < 0.002
    kp_eff = 0;
    ki_eff = 0;
    xi_a = 0;
    xi_b = 0;
    xi_c = 0;
    err_eff = 0;
elseif err_pu >= 0
    kp_eff = abs(vreg_kp);
    ki_eff = abs(vreg_ki);
    err_eff = err_pu;
else
    kp_eff = abs(vreg_kp) * swell_gain;
    ki_eff = abs(vreg_ki) * swell_gain;
    err_eff = err_pu;
    if kp_eff == 0 && ki_eff == 0
        xi_a = 0;
        xi_b = 0;
        xi_c = 0;
    end
end
if t_ctrl > 0.02
    xi_a = xi_a + ki_eff * err_eff * ts;
else
    xi_a = 0;
end
m_unsat = kp_eff * err_eff + xi_a;
m_cmd = min(max(m_unsat, -m_max), m_max);
if m_cmd ~= m_unsat
    xi_a = m_cmd - kp_eff * err_eff;
end
ma = m_cmd * sin(theta + phi);
mb = m_cmd * sin(theta + phi - 2*pi/3);
mc = m_cmd * sin(theta + phi + 2*pi/3);
m_amp = sqrt((ma*ma + mb*mb + mc*mc) / 3);
m_ref6 = [ma; -ma; mb; -mb; mc; -mc];
ctrl_dbg = [theta; vd; vq; v_meas; v_err; m_amp; phi];
end

== matlab function hpt_v2_1to1_switchlevel/HPTSACController/HPT_SAC_HLC ==
  data: Vlv input; m_reg6 output; Vdc input; Venergy input; Ienergy input; ts input; grid_f0 input; vref_phase input; vdc_ref input; policy_mode input; actor_select_mode input; reg_max input; energy_max input; i_base_peak input; inj_phase input; reg_polarity input; reg_d_gain input; reg_q_gain input; dynamic_reg_limit input; energy_polarity input; topology_id input; fixed_reg_d input; fixed_reg_q input; fixed_energy_d input; fixed_energy_q input; guard_enable input; energy_id_max input; energy_i_kp input; energy_i_ki input; energy_vff_gain input; energy_control_sign input; m_energy3 output; obs24 output; act4 output
function [m_reg6, m_energy3, obs24, act4] = fcn(Vlv, Vdc, Venergy, Ienergy, ts, grid_f0, vref_phase, vdc_ref, policy_mode, actor_select_mode, reg_max, energy_max, i_base_peak, inj_phase, reg_polarity, reg_d_gain, reg_q_gain, dynamic_reg_limit, energy_polarity, topology_id, fixed_reg_d, fixed_reg_q, fixed_energy_d, fixed_energy_q, guard_enable, energy_id_max, energy_i_kp, energy_i_ki, energy_vff_gain, energy_control_sign)
%#codegen
persistent theta xi_pll xi_eid xi_eiq ba bb bi v_rms_f last_act t_clock fault_active recovery_active fault_start_t dyn_fault_start_t dyn_fault_kind recovery_start_t v_fault_min v_fault_max last_vpos last_vdc normal_seen
if isempty(theta)
    theta = 0;
    xi_pll = 0;
    xi_eid = 0;
    xi_eiq = 0;
    ba = zeros(512,1);
    bb = zeros(512,1);
    bi = int32(1);
    v_rms_f = 0;
    last_act = zeros(4,1);
    t_clock = 0;
    fault_active = 0;
    recovery_active = 0;
    fault_start_t = 0;
    dyn_fault_start_t = 0;
    dyn_fault_kind = 0;
    recovery_start_t = 0;
    v_fault_min = 1;
    v_fault_max = 1;
    last_vpos = 1;
    last_vdc = 1;
    normal_seen = 0;
end
m_reg6 = zeros(6,1);
m_energy3 = zeros(3,1);
obs24 = zeros(24,1);
act4 = zeros(4,1);
t_clock = t_clock + ts;
va = Vlv(1); vb = Vlv(2); vc = Vlv(3);
alpha = (2/3) * (va - 0.5*vb - 0.5*vc);
beta = (sqrt(3)/3) * (vb - vc);
theta_meas = atan2(beta, alpha);
pll_err = atan2(sin(theta_meas - theta), cos(theta_meas - theta));
xi_pll = xi_pll + 1200 * pll_err * ts;
if xi_pll > 120; xi_pll = 120; elseif xi_pll < -120; xi_pll = -120; end
omega = 2*pi*grid_f0 + 70 * pll_err + xi_pll;
theta = theta + omega * ts;
theta = theta - 2*pi*floor(theta/(2*pi));
nb = int32(round(0.25 / max(grid_f0*ts, 1e-9)));
if nb < 1; nb = int32(1); elseif nb > 512; nb = int32(512); end
iad = ba(bi); ibd = bb(bi);
ba(bi) = alpha; bb(bi) = beta;
bi = bi + 1; if bi > nb; bi = int32(1); end
vbase_peak = sqrt(2) * max(vref_phase, 1);
v1a = 0.5*(alpha - ibd); v1b = 0.5*(beta + iad);
v2a = 0.5*(alpha + ibd); v2b = 0.5*(beta - iad);
vpos = sqrt(v1a*v1a + v1b*v1b) / vbase_peak;
vneg = sqrt(v2a*v2a + v2b*v2b) / vbase_peak;
v_rms = sqrt(max((va*va + vb*vb + vc*vc) / 3, 0));
if v_rms_f == 0; v_rms_f = v_rms; end
alpha_v = min(max(ts / 0.005, 0), 1);
v_rms_f = v_rms_f + alpha_v * (v_rms - v_rms_f);
vpu = v_rms_f / max(vref_phase, 1);
vdcpu = Vdc / max(vdc_ref, 1);
ea = Ienergy(1); eb = Ienergy(2); ec = Ienergy(3);
ialpha = (2/3) * (ea - 0.5*eb - 0.5*ec);
ibeta = (sqrt(3)/3) * (eb - ec);
ct = cos(theta); st = sin(theta);
id_e = (ialpha*ct + ibeta*st) / max(i_base_peak, 1);
iq_e = (-ialpha*st + ibeta*ct) / max(i_base_peak, 1);
reg_mag_prev = sqrt(last_act(1)*last_act(1) + last_act(2)*last_act(2));
energy_mag_prev = sqrt(last_act(3)*last_act(3) + last_act(4)*last_act(4));
measured_fault = double((vpos < 0.92) || (vpos > 1.08) || (vneg > 0.04));
normal_band = double((vpos >= 0.97) && (vpos <= 1.03) && (vneg <= 0.025));
if normal_band >= 0.5 && t_clock > 0.015
    normal_seen = 1;
end
if measured_fault >= 0.5
    if fault_active < 0.5
        fault_start_t = t_clock;
        if dyn_fault_start_t == 0 && t_clock > 0.02; dyn_fault_start_t = t_clock; if vpos > 1; dyn_fault_kind = 1; else; dyn_fault_kind = -1; end; end
        v_fault_min = vpos;
        v_fault_max = vpos;
    end
    fault_active = 1;
    recovery_active = 0;
    v_fault_min = min(v_fault_min, vpos);
    v_fault_max = max(v_fault_max, vpos);
    if dyn_fault_start_t > 0 && (t_clock - dyn_fault_start_t) < 0.02 && v_fault_min < 0.94; dyn_fault_kind = -1; end
    if dyn_fault_start_t > 0 && (t_clock - dyn_fault_start_t) < 0.02 && v_fault_min > 0.97 && vpos > 1.02; dyn_fault_kind = 1; end
    if dyn_fault_start_t > 0 && (t_clock - dyn_fault_start_t) < 0.03 && v_fault_min > 0.97 && vdcpu > 1.12; dyn_fault_kind = 1; end
elseif fault_active >= 0.5
    fault_active = 0;
    recovery_active = 1;
    recovery_start_t = t_clock;
elseif recovery_active >= 0.5 && normal_band >= 0.5 && (t_clock - recovery_start_t) >= 0.08
    recovery_active = 0;
    v_fault_min = 1;
    v_fault_max = 1;
end
tfault = 0; if fault_active >= 0.5; tfault = min(max((t_clock - fault_start_t)/0.5, 0), 1); end
trec = 0; if recovery_active >= 0.5; trec = min(max((t_clock - recovery_start_t)/0.5, 0), 1); end
dynamic_fault = double(dyn_fault_start_t > 0.02);
dvpos = (vpos - last_vpos) / max(ts, 1e-9) / 50;
dvdc = (vdcpu - last_vdc) / max(ts, 1e-9) / 50;
last_vpos = vpos;
last_vdc = vdcpu;
obs24 = [vpu; vpos; vneg; vdcpu; 1-vdcpu; 1-vpu; id_e; iq_e; last_act; double(vpos < 0.92); double(vpos > 1.08); double(topology_id < 1.5); double(topology_id >= 1.5); fault_active; recovery_active; tfault; trec; v_fault_min; v_fault_max; dvpos; dvdc];
for k=1:24; if obs24(k)>5; obs24(k)=5; elseif obs24(k)<-5; obs24(k)=-5; end; end
if policy_mode <= -0.5
    act4 = [fixed_reg_d; fixed_reg_q; fixed_energy_d; fixed_energy_q];
elseif policy_mode >= 0.5
    use_dynamic_actor = false;
    if actor_select_mode >= 1.5
        if dynamic_reg_limit < 0.90 * reg_max
            use_dynamic_actor = dynamic_fault >= 0.5;
        else
            use_dynamic_actor = true;
        end
    elseif actor_select_mode >= 0.5
        use_dynamic_actor = normal_seen >= 0.5 && t_clock > 0.02;
    end
    if use_dynamic_actor
        W = coder.load('hpt_sac_actor_weights_dynamic.mat');
    else
        W = coder.load('hpt_sac_actor_weights.mat');
    end
    H = 256; OBS_DIM = 24; N_ACT = 4;
    W0 = reshape(W.latent_pi_0_weight, H, OBS_DIM); b0 = reshape(W.latent_pi_0_bias, H, 1);
    W2 = reshape(W.latent_pi_2_weight, H, H); b2 = reshape(W.latent_pi_2_bias, H, 1);
    W4 = reshape(W.latent_pi_4_weight, H, H); b4 = reshape(W.latent_pi_4_bias, H, 1);
    Wm = reshape(W.mu_weight, N_ACT, H); bm = reshape(W.mu_bias, N_ACT, 1);
    alo = reshape(W.act_low, N_ACT, 1); ahi = reshape(W.act_high, N_ACT, 1);
    h = max(0, W0*obs24 + b0);
    h = max(0, W2*h + b2);
    h = max(0, W4*h + b4);
    mu = Wm*h + bm;
    act4 = alo + 0.5*(tanh(mu)+1).*(ahi-alo);
else
    act4 = zeros(4,1);
    if fault_active >= 0.5
        if vpos < 0.97
            if topology_id < 1.5
                act4(1) = 0.40; act4(2) = 0.00; act4(3) = 0.20; act4(4) = 0.00;
                if vpos < 0.78; act4(1) = 0.58; act4(3) = 0.10; end
            else
                act4(1) = 0.60; act4(2) = 0.00; act4(3) = 0.20; act4(4) = 0.00;
                if vpos < 0.78; act4(1) = 0.78; act4(3) = 0.00; end
            end
        elseif vpos > 1.03
            if topology_id < 1.5
                act4(1) = 0.00; act4(2) = 0.00; act4(3) = 0.00; act4(4) = 0.00;
            else
                act4(1) = 0.00; act4(2) = 0.00; act4(3) = -0.25; act4(4) = 0.00;
            end
        end
    end
end
if guard_enable >= 0.5
    if vpos < 0.92 && act4(1) < 0; act4(1) = 0; end
    if vpos > 1.08 && act4(1) > 0; act4(1) = 0; end
    if vpu < 0.98 && act4(1) < 0; act4(1) = 0; end
    if vdcpu < 0.95
        dc_scale = min(max((vdcpu - 0.75)/0.20, 0), 1);
        act4(1) = dc_scale * act4(1);
        act4(3) = max(act4(3), min(energy_max, 0.20 + 1.2*(0.82-vdcpu)));
    elseif vdcpu > 1.12
        act4(3) = min(act4(3), -0.05);
    end
end
if guard_enable >= 0.5 && policy_mode >= 0.5 && topology_id < 1.5 && actor_select_mode < 1.5
    top1_reg = 0.32 + 2.35*(1 - vpu);
    if vpu > 0.995; top1_reg = 0.26; end
    if top1_reg < 0.22; top1_reg = 0.22; elseif top1_reg > 0.46; top1_reg = 0.46; end
    act4(1) = top1_reg;
    act4(2) = 0;
    act4(3) = 0;
    act4(4) = 0;
end
if guard_enable >= 0.5 && policy_mode >= 0.5 && actor_select_mode >= 1.5 && topology_id >= 1.5
    dyn_lim0 = min(max(dynamic_reg_limit, 0), reg_max);
    dyn_cmd0 = 20.0 * (1 - vpu);
    if dyn_cmd0 > dyn_lim0; dyn_cmd0 = dyn_lim0; elseif dyn_cmd0 < -dyn_lim0; dyn_cmd0 = -dyn_lim0; end
    act4(1) = dyn_cmd0;
    act4(2) = 0;
    act4(3) = 0;
    act4(4) = 0;
end
if guard_enable >= 0.5 && actor_select_mode >= 1.5 && (dynamic_fault >= 0.5 && (fault_active >= 0.5 || recovery_active >= 0.5))
    dyn_lim = min(max(dynamic_reg_limit, 0), reg_max);
    if act4(1) > dyn_lim; act4(1) = dyn_lim; elseif act4(1) < -dyn_lim; act4(1) = -dyn_lim; end
    if act4(2) > dyn_lim; act4(2) = dyn_lim; elseif act4(2) < -dyn_lim; act4(2) = -dyn_lim; end
    if topology_id >= 1.5
        dyn_cmd = 20.0 * (1 - vpu);
        if dyn_cmd > dyn_lim; dyn_cmd = dyn_lim; elseif dyn_cmd < -dyn_lim; dyn_cmd = -dyn_lim; end
        act4(1) = dyn_cmd;
        act4(2) = 0;
        act4(3) = 0;
        act4(4) = 0;
    end
    if vpos < 0.92 && act4(1) < 0; act4(1) = 0; end
    if vpos > 1.08 && act4(1) > 0; act4(1) = 0; end
    if vpu < 0.98 && act4(1) < 0; act4(1) = 0; end
    if vdcpu < 0.95
        dc_scale = min(max((vdcpu - 0.75)/0.20, 0), 1);
        act4(1) = dc_scale * act4(1);
    end
end
act4(1) = min(max(act4(1), -reg_max), reg_max);
act4(2) = min(max(act4(2), -reg_max), reg_max);
act4(3) = min(max(act4(3), -energy_max), energy_max);
act4(4) = min(max(act4(4), -energy_max), energy_max);
md = reg_polarity * reg_d_gain * act4(1); mq = reg_polarity * reg_q_gain * act4(2);
phase_cmd = inj_phase;
if guard_enable >= 0.5 && topology_id >= 1.5 && actor_select_mode >= 1.5 && act4(1) < 0
    phase_cmd = inj_phase + 0.55;
end
pa = theta + phase_cmd;
pb = theta + phase_cmd - 2*pi/3;
pc = theta + phase_cmd + 2*pi/3;
ma = md*sin(pa) + mq*cos(pa);
mb = md*sin(pb) + mq*cos(pb);
mc = md*sin(pc) + mq*cos(pc);
m_reg6 = [ma; -ma; mb; -mb; mc; -mc];
eva = Venergy(1); evb = Venergy(2); evc = Venergy(3);
eia = Ienergy(1); eib = Ienergy(2); eic = Ienergy(3);
evalpha = (2/3) * (eva - 0.5*evb - 0.5*evc);
evbeta = (sqrt(3)/3) * (evb - evc);
eialpha = (2/3) * (eia - 0.5*eib - 0.5*eic);
eibeta = (sqrt(3)/3) * (eib - eic);
evd = evalpha*ct + evbeta*st;
evq = -evalpha*st + evbeta*ct;
eid = eialpha*ct + eibeta*st;
eiq = -eialpha*st + eibeta*ct;
eid_ref = energy_id_max * act4(3);
eiq_ref = energy_id_max * act4(4);
eeid = eid_ref - eid;
eeiq = eiq_ref - eiq;
xi_eid = xi_eid + energy_i_ki * eeid * ts;
xi_eiq = xi_eiq + energy_i_ki * eeiq * ts;
ed_ctrl = energy_i_kp * eeid + xi_eid;
eq_ctrl = energy_i_kp * eeiq + xi_eiq;
evconv_d = energy_vff_gain * evd - energy_control_sign * ed_ctrl;
evconv_q = energy_vff_gain * evq - energy_control_sign * eq_ctrl;
econv_alpha = evconv_d*ct - evconv_q*st;
econv_beta = evconv_d*st + evconv_q*ct;
ema_unsat = 2 * econv_alpha / max(abs(Vdc), 50);
emb_unsat = 2 * (-0.5*econv_alpha + (sqrt(3)/2)*econv_beta) / max(abs(Vdc), 50);
emc_unsat = 2 * (-0.5*econv_alpha - (sqrt(3)/2)*econv_beta) / max(abs(Vdc), 50);
ema = min(max(ema_unsat, -energy_max), energy_max);
emb = min(max(emb_unsat, -energy_max), energy_max);
emc = min(max(emc_unsat, -energy_max), energy_max);
if abs(ema) >= energy_max || abs(emb) >= energy_max || abs(emc) >= energy_max
    xi_eid = xi_eid - energy_i_ki * eeid * ts;
    xi_eiq = xi_eiq - energy_i_ki * eeiq * ts;
end
m_energy3 = energy_polarity * [ema; emb; emc];
last_act = act4;
end
